simulink subsystem "lat_deg_to_km"  (R2022a)
settings: Solver=VariableStepAuto  StartTime=0.0  StopTime=10.0  RelTol=1e-3
settings Model: Creator=rodri  LastModifiedBy=rodri

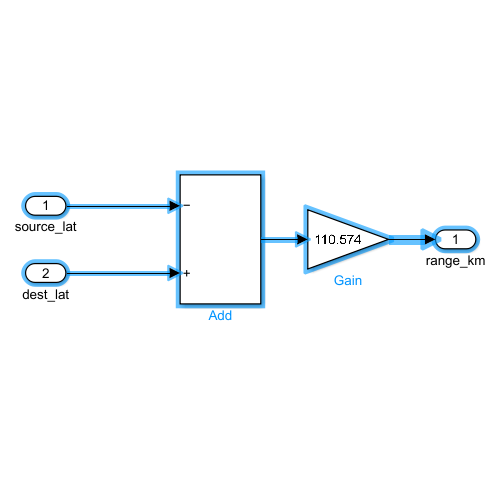
[thumbnail: Simulink's stored preview of the top-level diagram]
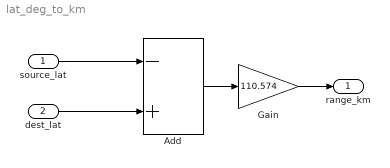
== system lat_deg_to_km ==
  source_lat : Inport
  dest_lat : Inport  Port=2
  Add : Sum  Inputs=-+
  Gain : Gain  Gain=110.574
  range_km : Outport
  wires:
  source_lat/1 -> Add/1
  Add/1 -> Gain/1
  dest_lat/1 -> Add/2
  Gain/1 -> range_km/1
